simulink model "motor_control_with_homebrew_SVPWM"  (Simulink 7.9)
settings: Solver=ode45  StartTime=0.0  StopTime=1  RelTol=1e-3
libraries: powerlib x17, simulink x6
settings Model: Creator=Dmitriy  LastModifiedBy=Dmitriy
settings GRTTargetCC: CombineOutputUpdateFcns=off  GRTInterface=on

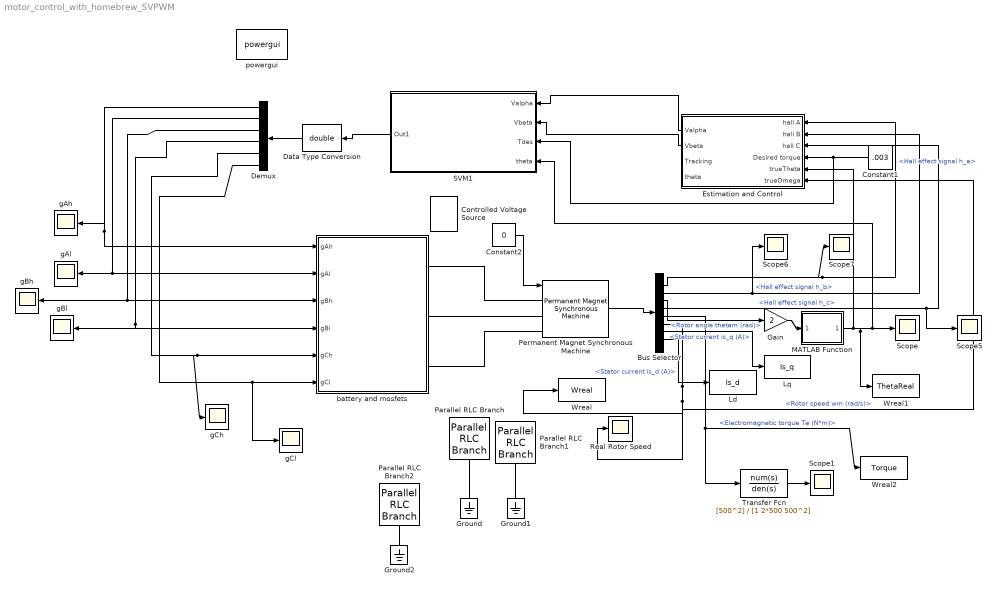
== system motor_control_with_homebrew_SVPWM ==
  Bus Selector : BusSelector  OutputSignals=Hall effect signal h_a,Hall effect signal h_b,Hall effect signal h_c,Rotor angle thetam (rad),Electromagnetic torque Te (N*m),Rotor speed wm (rad/s),Stator current is_q (A),Stator current is_d (A)
  Constant1 : Constant  Value=.003
  Constant2 : Constant  Value=0
  Controlled Voltage Source : powerlib/Electrical Sources/Controlled Voltage Source  Initialize=on  Source_Type=AC  Amplitude=0  Phase=0  Frequency=0  Measurements=None
  Data Type Conversion : DataTypeConversion  OutDataTypeStr=double
  Demux : Demux  Outputs=6
  Estimation and Control : Subsystem  SystemSampleTime=.001
  Gain : Gain  Gain=2
  Ground : powerlib/Elements/Ground  LConnTagsString=a
  Ground1 : powerlib/Elements/Ground  LConnTagsString=a
  Ground2 : powerlib/Elements/Ground  LConnTagsString=a
  Ld : ToWorkspace  VariableName=Is_d  SampleTime=-1  SaveFormat=Timeseries
  Lq : ToWorkspace  VariableName=Is_q  SampleTime=-1  SaveFormat=Timeseries
  MATLAB Function : MATLAB Function  TreatAsAtomicUnit=on
  Parallel RLC Branch : powerlib/Elements/Parallel RLC Branch  LConnTagsString=a  RConnTagsString=__new0  BranchType=RC  Resistance=100000  Inductance=1e-3  SetiL0=off  InitialCurrent=0  Capacitance=1e-4  Setx0=off  InitialVoltage=0  Measurements=None
  Parallel RLC Branch1 : powerlib/Elements/Parallel RLC Branch  LConnTagsString=a  RConnTagsString=__new0  BranchType=RC  Resistance=100000  Inductance=1e-3  SetiL0=off  InitialCurrent=0  Capacitance=1e-4  Setx0=off  InitialVoltage=0  Measurements=None
  Parallel RLC Branch2 : powerlib/Elements/Parallel RLC Branch  LConnTagsString=a  RConnTagsString=__new0  BranchType=RC  Resistance=100000  Inductance=1e-3  SetiL0=off  InitialCurrent=0  Capacitance=1e-4  Setx0=off  InitialVoltage=0  Measurements=None
  Permanent Magnet Synchronous Machine : powerlib/Machines/Permanent Magnet Synchronous Machine  NbPhases=3  FluxDistribution=Sinusoidal  RotorType=Round  MechanicalLoad=Torque Tm  PresetModel=No  ShowDetailedParameters=on  Resistance=28.2  Inductance=8.5e-3  dqInductances=[0.006365 0.006365]  La=1940*10^-6  MachineConstant=Torque Constant (N.m / A_peak)  Flux=0.005225  VoltageCst=1.8954  TorqueCst=0.0181*sqrt(3)/2  Flat=120  Mechanical=[0.0001 5.396e-005 2 0]  PolePairs=2  InitialConditions=[0,1, 0,0]  InitialConditions5ph=[0 0 0 0 0 0]  TsPowergui=0  TsBlock=-1  RefAngle=Aligned with phase A axis (original Park)
  Real Rotor Speed : Scope
      settings: YMin=9.27  YMax=9.44  SaveName=ScopeData18
  SVM1 : Subsystem  SystemSampleTime=10^-6
  Scope{,1,5..7} (5 alike) : Scope
      Scope settings: YMin=0.03925  YMax=0.0396
      Scope1 settings: YMin=0.0028  YMax=0.003275
      Scope5 settings: SaveName=ScopeData5
      Scope6 settings: SaveName=ScopeData6
      Scope7 settings: SaveName=ScopeData7
  Transfer Fcn : TransferFcn  Numerator=[500^2]  Denominator=[1 2*500 500^2]
  Wreal : ToWorkspace  VariableName=Wreal  SampleTime=-1  SaveFormat=Timeseries
  Wreal1 : ToWorkspace  VariableName=ThetaReal  SampleTime=-1  SaveFormat=Timeseries
  Wreal2 : ToWorkspace  VariableName=Torque  SampleTime=-1  SaveFormat=Timeseries
  battery and mosfets : Subsystem
  gAh : Scope
      settings: SaveName=ScopeData11
  gAl : Scope
      settings: SaveName=ScopeData10
  gBh : Scope
      settings: SaveName=ScopeData9
  gBl : Scope
      settings: YMin=0.998725  YMax=0.99925  SaveName=ScopeData8
  gCh : Scope
      settings: YMin=0.95  YMax=1.05  SaveName=ScopeData4
  gCl : Scope
      settings: YMin=0.95  YMax=1.05  SaveName=ScopeData2
  powergui : powerlib/powergui  Priority=1  SimulationMode=Discrete  SolverType=Tustin  SampleTime=1e-6  frequency=60  SPID=off  DisableSnubberDevices=off  DisableRonSwitches=off  DisableVfSwitches=off  SwTol=0  Interpol=off  DisplayEquations=off  FunctionMessages=off  frequencyindice=0  Pbase=100e6  ErrMax=1e-4  Iterations=50  UnitsV=kV  UnitsW=MW  echomessages=off  HookPort=off  EnableUseOfTLC=off  x0status=blocks  RestoreLinks=warning  ResistiveCurrentMeasurement=off  Ylog=off  Xlog=on  ShowGrid=off  save=off  variable=ZData  ZoomFFT=off  StartTime=0.0  cycles=1  DisplayStyle=1  FreqAxis=off  MaxFrequency=1000  frequencyindicesteady=1  display=off  methode=off
  wires:
  Permanent Magnet Synchronous Machine/1 -> Bus Selector/1
  Bus Selector/1 -> Estimation and Control/1(hall A), Scope7/1  "<Hall effect signal h_a>"
  Bus Selector/3 -> Estimation and Control/3(hall C), Scope5/1  "<Hall effect signal h_c>"
  Bus Selector/4 -> Gain/1  "<Rotor angle thetam (rad)>"
  Bus Selector/5 -> Wreal2/1, Transfer Fcn/1  "<Electromagnetic torque Te (N*m)>"
  Bus Selector/2 -> Estimation and Control/2(hall B), Scope6/1  "<Hall effect signal h_b>"
  Demux/6 -> battery and mosfets/6(gCl), gCl/1
  Demux/5 -> battery and mosfets/5(gCh), gCh/1
  Demux/4 -> battery and mosfets/4(gBl), gBl/1
  Demux/3 -> battery and mosfets/3(gBh), gBh/1
  Demux/2 -> battery and mosfets/2(gAl), gAl/1
  Demux/1 -> battery and mosfets/1(gAh), gAh/1
  Constant1/1 -> Estimation and Control/4(Desired torque), SVM1/3(Tdes)
  Bus Selector/6 -> Real Rotor Speed/1, Wreal/1, Estimation and Control/6(trueOmega)  "<Rotor speed wm (rad/s)>"
  MATLAB Function/1(lambda1) -> Wreal1/1, Scope/1, SVM1/4(theta), Estimation and Control/5(trueTheta)
  Gain/1 -> MATLAB Function/1(lambda)
  Constant2/1 -> Permanent Magnet Synchronous Machine/1
  Estimation and Control/1(Valpha) -> SVM1/1(Valpha)
  Estimation and Control/2(Vbeta) -> SVM1/2(Vbeta)
  SVM1/1(Out1) -> Data Type Conversion/1
  Bus Selector/7 -> Lq/1  "<Stator current is_q (A)>"
  Bus Selector/8 -> Ld/1  "<Stator current is_d (A)>"
  Transfer Fcn/1 -> Scope1/1
  Data Type Conversion/1 -> Demux/1
  connections:
  Permanent Magnet Synchronous Machine/LConn1 -- battery and mosfets/RConn1
  battery and mosfets/RConn2 -- Permanent Magnet Synchronous Machine/LConn2
  Permanent Magnet Synchronous Machine/LConn3 -- battery and mosfets/RConn3
  Parallel RLC Branch/RConn1 -- Ground/LConn1
  Ground1/LConn1 -- Parallel RLC Branch1/RConn1
  Parallel RLC Branch2/RConn1 -- Ground2/LConn1

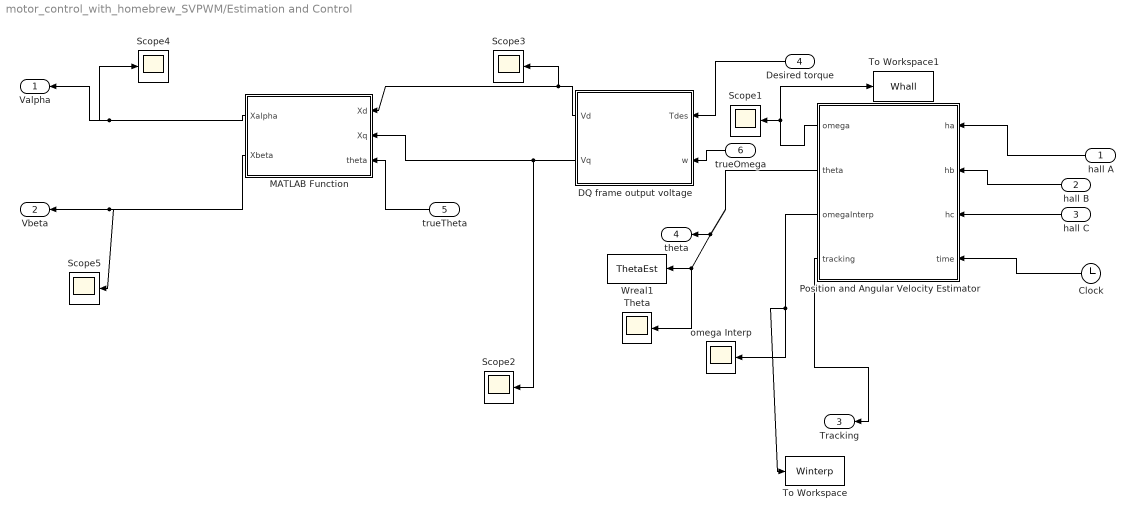
== system motor_control_with_homebrew_SVPWM/Estimation and Control ==
  hall A : Inport
  hall B : Inport  Port=2
  hall C : Inport  Port=3
  Desired torque : Inport  Port=4
  trueTheta : Inport  Port=5
  trueOmega : Inport  Port=6
  Clock : Clock
  DQ frame output voltage : MATLAB Function  TreatAsAtomicUnit=on  SystemSampleTime=.0001
  MATLAB Function : MATLAB Function  TreatAsAtomicUnit=on
  Position and Angular Velocity Estimator : MATLAB Function  TreatAsAtomicUnit=on  SystemSampleTime=.0001
  Scope{1..5} (5 alike) : Scope
      Scope1 settings: SaveName=ScopeData13
      Scope2 settings: YMin=4.67403  YMax=4.67403  SaveName=ScopeData14
      Scope3 settings: SaveName=ScopeData15
      Scope4 settings: SaveName=ScopeData16
      Scope5 settings: SaveName=ScopeData17
  Theta : Scope
      settings: YMin=5.75959  YMax=5.75959  SaveName=ScopeData12
  To Workspace : ToWorkspace  VariableName=Winterp  SampleTime=-1  SaveFormat=Timeseries
  To Workspace1 : ToWorkspace  VariableName=Whall  SampleTime=-1  SaveFormat=Timeseries
  Wreal1 : ToWorkspace  VariableName=ThetaEst  SampleTime=-1  SaveFormat=Timeseries
  omega Interp : Scope
      settings: YMin=0  YMax=3.25  SaveName=ScopeData19
  Valpha : Outport
  Vbeta : Outport  Port=2
  Tracking : Outport  Port=3
  theta : Outport  Port=4
  wires:
  Position and Angular Velocity Estimator/1(omega) -> Scope1/1, To Workspace1/1
  Desired torque/1 -> DQ frame output voltage/1(Tdes)
  hall A/1 -> Position and Angular Velocity Estimator/1(ha)
  hall B/1 -> Position and Angular Velocity Estimator/2(hb)
  hall C/1 -> Position and Angular Velocity Estimator/3(hc)
  Position and Angular Velocity Estimator/2(theta) -> Theta/1, Wreal1/1, theta/1
  DQ frame output voltage/2(Vq) -> Scope2/1, MATLAB Function/2(Xq)
  DQ frame output voltage/1(Vd) -> Scope3/1, MATLAB Function/1(Xd)
  MATLAB Function/1(Xalpha) -> Valpha/1, Scope4/1
  MATLAB Function/2(Xbeta) -> Vbeta/1, Scope5/1
  Position and Angular Velocity Estimator/3(omegaInterp) -> omega Interp/1, To Workspace/1
  Clock/1 -> Position and Angular Velocity Estimator/4(time)
  Position and Angular Velocity Estimator/4(tracking) -> Tracking/1
  trueTheta/1 -> MATLAB Function/3(theta)
  trueOmega/1 -> DQ frame output voltage/2(w)

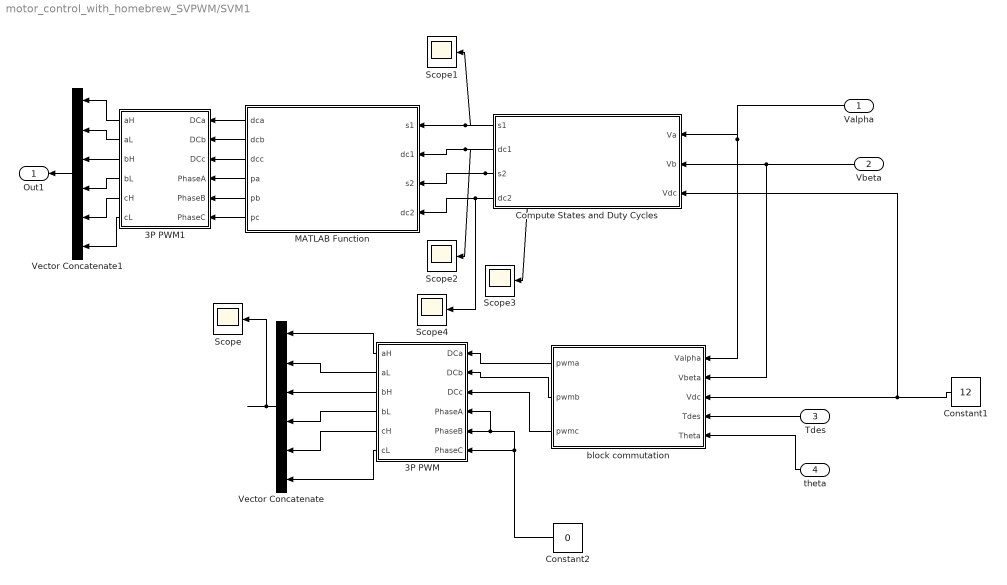
== system motor_control_with_homebrew_SVPWM/SVM1 ==
  Valpha : Inport
  Vbeta : Inport  Port=2
  Tdes : Inport  Port=3
  theta : Inport  Port=4
  3P PWM : Subsystem  TreatAsAtomicUnit=on  SystemSampleTime=1
  3P PWM1 : Subsystem  TreatAsAtomicUnit=on  SystemSampleTime=10^-6
  Compute States and Duty Cycles : MATLAB Function  TreatAsAtomicUnit=on  SystemSampleTime=.001
  Constant1 : Constant  Value=12
  Constant2 : Constant  Value=0
  MATLAB Function : MATLAB Function  TreatAsAtomicUnit=on  SystemSampleTime=10^-6
  Scope{,1..4} (5 alike) : Scope
      Scope settings: SaveName=ScopeData3
      Scope1 settings: SaveName=ScopeData6
      Scope2 settings: SaveName=ScopeData7
      Scope3 settings: SaveName=ScopeData8
      Scope4 settings: SaveName=ScopeData9
  Vector Concatenate : Concatenate  NumInputs=6
  Vector Concatenate1 : Concatenate  NumInputs=6
  block commutation : MATLAB Function  TreatAsAtomicUnit=on  SystemSampleTime=1
  Out1 : Outport
  wires:
  Valpha/1 -> block commutation/1(Valpha), Compute States and Duty Cycles/1(Va)
  Vbeta/1 -> block commutation/2(Vbeta), Compute States and Duty Cycles/2(Vb)
  Constant1/1 -> block commutation/3(Vdc), Compute States and Duty Cycles/3(Vdc)
  Tdes/1 -> block commutation/4(Tdes)
  theta/1 -> block commutation/5(Theta)
  block commutation/2(pwmb) -> 3P PWM/2(DCb)
  block commutation/3(pwmc) -> 3P PWM/3(DCc)
  block commutation/1(pwma) -> 3P PWM/1(DCa)
  3P PWM/1(aH) -> Vector Concatenate/1
  3P PWM/2(aL) -> Vector Concatenate/2
  3P PWM/3(bH) -> Vector Concatenate/3
  3P PWM/4(bL) -> Vector Concatenate/4
  3P PWM/5(cH) -> Vector Concatenate/5
  3P PWM/6(cL) -> Vector Concatenate/6
  Vector Concatenate/1 -> Scope/1
  Constant2/1 -> 3P PWM/6(PhaseC), 3P PWM/5(PhaseB), 3P PWM/4(PhaseA)
  MATLAB Function/1(dca) -> 3P PWM1/1(DCa)
  MATLAB Function/2(dcb) -> 3P PWM1/2(DCb)
  MATLAB Function/3(dcc) -> 3P PWM1/3(DCc)
  MATLAB Function/4(pa) -> 3P PWM1/4(PhaseA)
  MATLAB Function/5(pb) -> 3P PWM1/5(PhaseB)
  MATLAB Function/6(pc) -> 3P PWM1/6(PhaseC)
  3P PWM1/1(aH) -> Vector Concatenate1/1
  3P PWM1/2(aL) -> Vector Concatenate1/2
  3P PWM1/3(bH) -> Vector Concatenate1/3
  3P PWM1/4(bL) -> Vector Concatenate1/4
  3P PWM1/5(cH) -> Vector Concatenate1/5
  3P PWM1/6(cL) -> Vector Concatenate1/6
  Compute States and Duty Cycles/1(s1) -> MATLAB Function/1(s1), Scope1/1
  Compute States and Duty Cycles/2(dc1) -> MATLAB Function/2(dc1), Scope2/1
  Compute States and Duty Cycles/3(s2) -> MATLAB Function/3(s2), Scope3/1
  Compute States and Duty Cycles/4(dc2) -> MATLAB Function/4(dc2), Scope4/1
  Vector Concatenate1/1 -> Out1/1

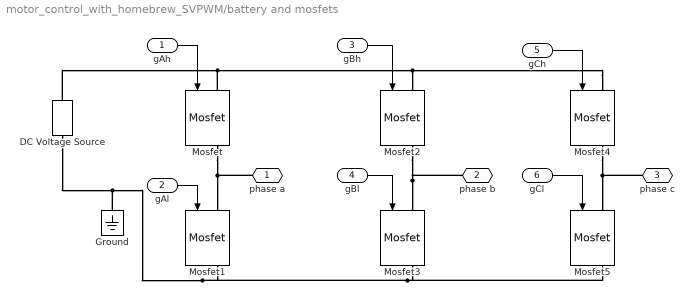
== system motor_control_with_homebrew_SVPWM/battery and mosfets ==
  gAh : Inport
  gAl : Inport  Port=2
  gBh : Inport  Port=3
  gBl : Inport  Port=4
  gCh : Inport  Port=5
  gCl : Inport  Port=6
  DC Voltage Source : powerlib/Electrical Sources/DC Voltage Source  Amplitude=12  Measurements=None
  Ground : powerlib/Elements/Ground  LConnTagsString=a
  Mosfet{,1..5} (6 alike) : powerlib/Power Electronics/Mosfet  Ron=0.1  Lon=0  Rd=0.01  Vfd=0  IC=0  Rs=1e5  Cs=inf  Measurements=on
  phase a : PMIOPort  Port=1  Side=Right
  phase b : PMIOPort  Port=2  Side=Right
  phase c : PMIOPort  Port=3  Side=Right
  wires:
  gCl/1 -> Mosfet5/1
  gCh/1 -> Mosfet4/1
  gBh/1 -> Mosfet2/1
  gBl/1 -> Mosfet3/1
  gAl/1 -> Mosfet1/1
  gAh/1 -> Mosfet/1
  connections:
  Mosfet/RConn1 -- Mosfet1/LConn1 -- phase a/RConn1
  Mosfet2/RConn1 -- Mosfet3/LConn1 -- phase b/RConn1
  phase c/RConn1 -- Mosfet4/RConn1 -- Mosfet5/LConn1
  Mosfet1/RConn1 -- Ground/LConn1 -- DC Voltage Source/LConn1 -- Mosfet3/RConn1 -- Mosfet5/RConn1
  Mosfet4/LConn1 -- Mosfet/LConn1 -- DC Voltage Source/RConn1 -- Mosfet2/LConn1

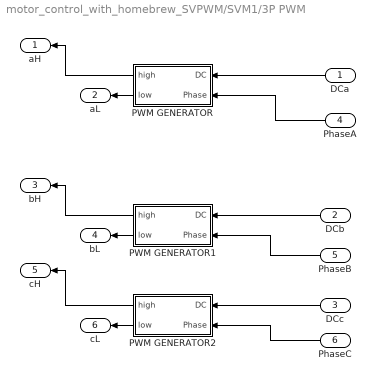
== system motor_control_with_homebrew_SVPWM/SVM1/3P PWM ==
  DCa : Inport
  DCb : Inport  Port=2
  DCc : Inport  Port=3
  PhaseA : Inport  Port=4
  PhaseB : Inport  Port=5
  PhaseC : Inport  Port=6
  PWM GENERATOR : Subsystem  TreatAsAtomicUnit=on
      settings: ErrorFcn=10^6
  PWM GENERATOR1 : Subsystem  TreatAsAtomicUnit=on
  PWM GENERATOR2 : Subsystem  TreatAsAtomicUnit=on
  aH : Outport
  aL : Outport  Port=2
  bH : Outport  Port=3
  bL : Outport  Port=4
  cH : Outport  Port=5
  cL : Outport  Port=6
  wires:
  DCa/1 -> PWM GENERATOR/1(DC)
  PWM GENERATOR/1(high) -> aH/1
  PWM GENERATOR/2(low) -> aL/1
  DCb/1 -> PWM GENERATOR1/1(DC)
  PWM GENERATOR1/1(high) -> bH/1
  PWM GENERATOR1/2(low) -> bL/1
  DCc/1 -> PWM GENERATOR2/1(DC)
  PWM GENERATOR2/1(high) -> cH/1
  PWM GENERATOR2/2(low) -> cL/1
  PhaseA/1 -> PWM GENERATOR/2(Phase)
  PhaseB/1 -> PWM GENERATOR1/2(Phase)
  PhaseC/1 -> PWM GENERATOR2/2(Phase)

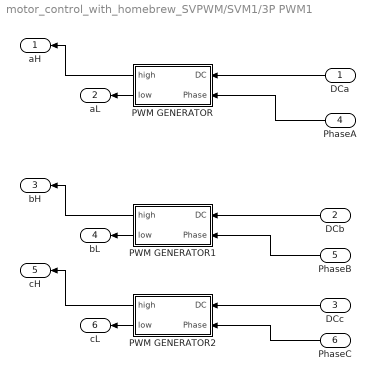
== system motor_control_with_homebrew_SVPWM/SVM1/3P PWM1 ==
  DCa : Inport
  DCb : Inport  Port=2
  DCc : Inport  Port=3
  PhaseA : Inport  Port=4
  PhaseB : Inport  Port=5
  PhaseC : Inport  Port=6
  PWM GENERATOR : Subsystem  TreatAsAtomicUnit=on
      settings: ErrorFcn=10^6
  PWM GENERATOR1 : Subsystem  TreatAsAtomicUnit=on
  PWM GENERATOR2 : Subsystem  TreatAsAtomicUnit=on
  aH : Outport
  aL : Outport  Port=2
  bH : Outport  Port=3
  bL : Outport  Port=4
  cH : Outport  Port=5
  cL : Outport  Port=6
  wires:
  DCa/1 -> PWM GENERATOR/1(DC)
  PWM GENERATOR/1(high) -> aH/1
  PWM GENERATOR/2(low) -> aL/1
  DCb/1 -> PWM GENERATOR1/1(DC)
  PWM GENERATOR1/1(high) -> bH/1
  PWM GENERATOR1/2(low) -> bL/1
  DCc/1 -> PWM GENERATOR2/1(DC)
  PWM GENERATOR2/1(high) -> cH/1
  PWM GENERATOR2/2(low) -> cL/1
  PhaseA/1 -> PWM GENERATOR/2(Phase)
  PhaseB/1 -> PWM GENERATOR1/2(Phase)
  PhaseC/1 -> PWM GENERATOR2/2(Phase)

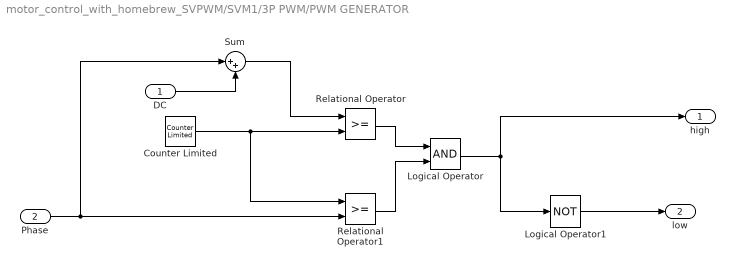
== system motor_control_with_homebrew_SVPWM/SVM1/3P PWM/PWM GENERATOR ==
  DC : Inport
  Phase : Inport  Port=2
  Counter Limited : simulink/Sources/Counter Limited  uplimit=1000  tsamp=-1
  Logical Operator : Logic  AllPortsSameDT=off  OutDataTypeStr=boolean
  Logical Operator1 : Logic  Operator=NOT  AllPortsSameDT=off  OutDataTypeStr=boolean
  Relational Operator : RelationalOperator  OutDataTypeStr=boolean
  Relational Operator1 : RelationalOperator  OutDataTypeStr=boolean
  Sum : Sum  Inputs=|++
  high : Outport
  low : Outport  Port=2
  wires:
  Counter Limited/1 -> Relational Operator/2, Relational Operator1/1
  Phase/1 -> Relational Operator1/2, Sum/1
  DC/1 -> Sum/2
  Sum/1 -> Relational Operator/1
  Relational Operator/1 -> Logical Operator/1
  Relational Operator1/1 -> Logical Operator/2
  Logical Operator/1 -> Logical Operator1/1, high/1
  Logical Operator1/1 -> low/1

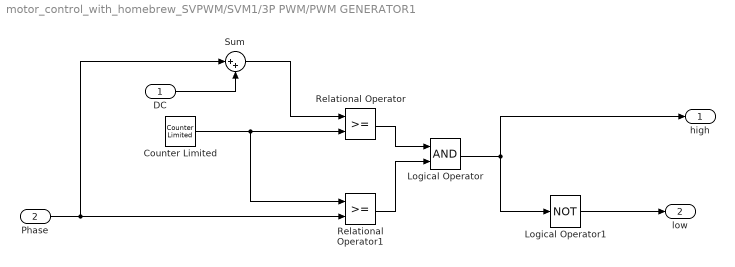
== system motor_control_with_homebrew_SVPWM/SVM1/3P PWM/PWM GENERATOR1 ==
  DC : Inport
  Phase : Inport  Port=2
  Counter Limited : simulink/Sources/Counter Limited  uplimit=1000  tsamp=-1
  Logical Operator : Logic  AllPortsSameDT=off  OutDataTypeStr=boolean
  Logical Operator1 : Logic  Operator=NOT  AllPortsSameDT=off  OutDataTypeStr=boolean
  Relational Operator : RelationalOperator  OutDataTypeStr=boolean
  Relational Operator1 : RelationalOperator  OutDataTypeStr=boolean
  Sum : Sum  Inputs=|++
  high : Outport
  low : Outport  Port=2
  wires:
  Counter Limited/1 -> Relational Operator/2, Relational Operator1/1
  Phase/1 -> Relational Operator1/2, Sum/1
  DC/1 -> Sum/2
  Sum/1 -> Relational Operator/1
  Relational Operator/1 -> Logical Operator/1
  Relational Operator1/1 -> Logical Operator/2
  Logical Operator/1 -> Logical Operator1/1, high/1
  Logical Operator1/1 -> low/1

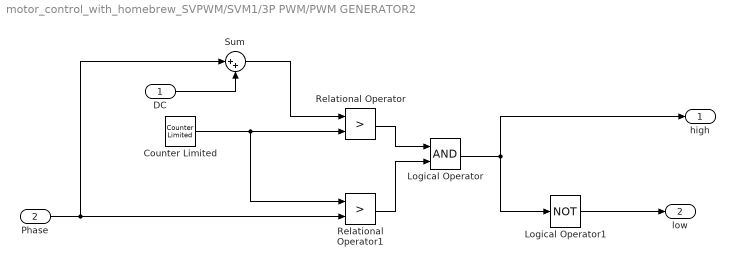
== system motor_control_with_homebrew_SVPWM/SVM1/3P PWM/PWM GENERATOR2 ==
  DC : Inport
  Phase : Inport  Port=2
  Counter Limited : simulink/Sources/Counter Limited  uplimit=1000  tsamp=-1
  Logical Operator : Logic  AllPortsSameDT=off  OutDataTypeStr=boolean
  Logical Operator1 : Logic  Operator=NOT  AllPortsSameDT=off  OutDataTypeStr=boolean
  Relational Operator : RelationalOperator  Operator=>  OutDataTypeStr=boolean
  Relational Operator1 : RelationalOperator  Operator=>  OutDataTypeStr=boolean
  Sum : Sum  Inputs=|++
  high : Outport
  low : Outport  Port=2
  wires:
  Counter Limited/1 -> Relational Operator/2, Relational Operator1/1
  Phase/1 -> Relational Operator1/2, Sum/1
  DC/1 -> Sum/2
  Sum/1 -> Relational Operator/1
  Relational Operator/1 -> Logical Operator/1
  Relational Operator1/1 -> Logical Operator/2
  Logical Operator/1 -> Logical Operator1/1, high/1
  Logical Operator1/1 -> low/1

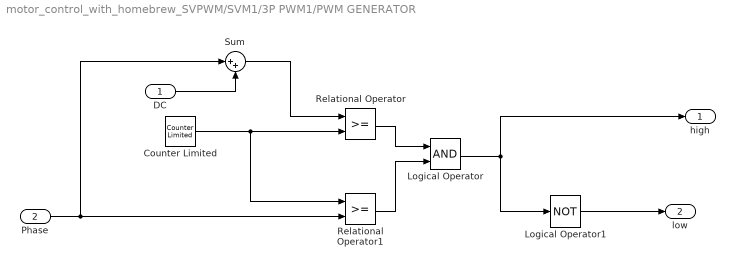
== system motor_control_with_homebrew_SVPWM/SVM1/3P PWM1/PWM GENERATOR ==
  DC : Inport
  Phase : Inport  Port=2
  Counter Limited : simulink/Sources/Counter Limited  uplimit=1000  tsamp=-1
  Logical Operator : Logic  AllPortsSameDT=off  OutDataTypeStr=boolean
  Logical Operator1 : Logic  Operator=NOT  AllPortsSameDT=off  OutDataTypeStr=boolean
  Relational Operator : RelationalOperator  OutDataTypeStr=boolean
  Relational Operator1 : RelationalOperator  OutDataTypeStr=boolean
  Sum : Sum  Inputs=|++
  high : Outport
  low : Outport  Port=2
  wires:
  Counter Limited/1 -> Relational Operator/2, Relational Operator1/1
  Phase/1 -> Relational Operator1/2, Sum/1
  DC/1 -> Sum/2
  Sum/1 -> Relational Operator/1
  Relational Operator/1 -> Logical Operator/1
  Relational Operator1/1 -> Logical Operator/2
  Logical Operator/1 -> Logical Operator1/1, high/1
  Logical Operator1/1 -> low/1

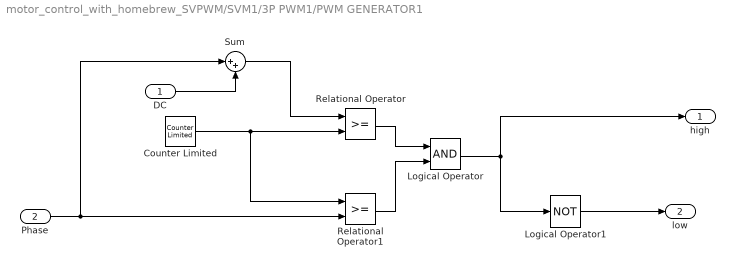
== system motor_control_with_homebrew_SVPWM/SVM1/3P PWM1/PWM GENERATOR1 ==
  DC : Inport
  Phase : Inport  Port=2
  Counter Limited : simulink/Sources/Counter Limited  uplimit=1000  tsamp=-1
  Logical Operator : Logic  AllPortsSameDT=off  OutDataTypeStr=boolean
  Logical Operator1 : Logic  Operator=NOT  AllPortsSameDT=off  OutDataTypeStr=boolean
  Relational Operator : RelationalOperator  OutDataTypeStr=boolean
  Relational Operator1 : RelationalOperator  OutDataTypeStr=boolean
  Sum : Sum  Inputs=|++
  high : Outport
  low : Outport  Port=2
  wires:
  Counter Limited/1 -> Relational Operator/2, Relational Operator1/1
  Phase/1 -> Relational Operator1/2, Sum/1
  DC/1 -> Sum/2
  Sum/1 -> Relational Operator/1
  Relational Operator/1 -> Logical Operator/1
  Relational Operator1/1 -> Logical Operator/2
  Logical Operator/1 -> Logical Operator1/1, high/1
  Logical Operator1/1 -> low/1

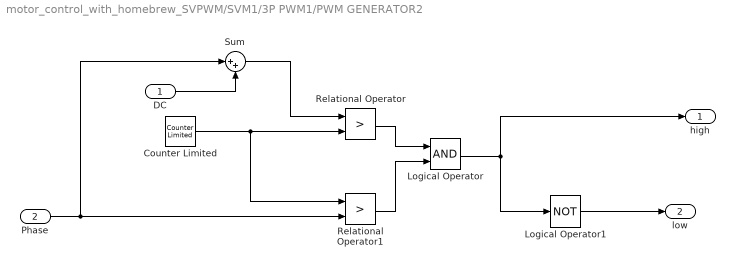
== system motor_control_with_homebrew_SVPWM/SVM1/3P PWM1/PWM GENERATOR2 ==
  DC : Inport
  Phase : Inport  Port=2
  Counter Limited : simulink/Sources/Counter Limited  uplimit=1000  tsamp=-1
  Logical Operator : Logic  AllPortsSameDT=off  OutDataTypeStr=boolean
  Logical Operator1 : Logic  Operator=NOT  AllPortsSameDT=off  OutDataTypeStr=boolean
  Relational Operator : RelationalOperator  Operator=>  OutDataTypeStr=boolean
  Relational Operator1 : RelationalOperator  Operator=>  OutDataTypeStr=boolean
  Sum : Sum  Inputs=|++
  high : Outport
  low : Outport  Port=2
  wires:
  Counter Limited/1 -> Relational Operator/2, Relational Operator1/1
  Phase/1 -> Relational Operator1/2, Sum/1
  DC/1 -> Sum/2
  Sum/1 -> Relational Operator/1
  Relational Operator/1 -> Logical Operator/1
  Relational Operator1/1 -> Logical Operator/2
  Logical Operator/1 -> Logical Operator1/1, high/1
  Logical Operator1/1 -> low/1

== matlab function Estimation and Control/DQ frame output voltage ==
  data: Tdes input double; Vd output double; w input double; Vq output double
function [Vd,Vq] = computeDQOutput(Tdes,w)
%#codegen
%take the desired torque current 
% speed and compute the output voltage vector in the DQ
%frame. 

L = 1940*10^-6*sqrt(3)/2;
R = 28.2;
Ke = (1.895*10^-3)*9.54929659643; % convert to V/(rad/s) 
Kt = 18.1*10^-3*sqrt(3)/2; %Nm/Amp
Ke = Kt;

%because I is assumed to be on Q axis, T = KtI
Ides = Tdes/Kt

%bemf is on q axis
bemf = Ke*w

%inductor impedance 
ZL = L*w;

Vq = (bemf+Ides*R)*3/2
Vd = (-ZL*Ides)*3/2

== matlab function Estimation and Control/Position and Angular Velocity Estimator ==
  data: omega output double; ha input double; theta output double; hb input double; hc input double; omegaInterp output double; time input double; tracking output double
function [omega,theta, omegaInterp, tracking] = rotor_est(ha,hb,hc,time)
%#codegen

%estimate the position of the rotor in degrees electrical
%tracking is 0 or 1, 0 means the estimate is bad. Used for activating block
%commutation at initialization
omega=0;
theta=0;
omegaInterp = 0;
time
tracking =0;
coder.extrinsic('rotor_estimate');

[omega theta omegaInterp tracking] = rotor_estimate(ha,hb,hc,time);
end

== matlab function MATLAB Function ==
  data: lambda input double; lambda1 output double
function lambda1 = wrapTo2Pi(lambda)
%wrapTo2Pi Wrap angle in radians to [0 2*pi]
%
%   lambdaWrapped = wrapTo2Pi(LAMBDA) wraps angles in LAMBDA, in radians,
%   to the interval [0 2*pi] such that zero maps to zero and 2*pi maps
%   to 2*pi. (In general, positive multiples of 2*pi map to 2*pi and
%   negative multiples of 2*pi map to zero.)
%
%   See also wrapToPi, wrapTo180, wrapTo360.

% Copyright 2007-2008 The MathWorks, Inc.
% $Revision: 1.1.6.1 $  $Date: 2008/12/22 23:50:53 $


positiveInput = (lambda > 0);
lambda = mod(lambda, 2*pi);
lambda((lambda == 0) & positiveInput) = 2*pi;
lambda1=lambda;
end

== matlab function Estimation and Control/MATLAB Function ==
  data: Xd input double; Xalpha output double; Xq input double; theta input double; Xbeta output double
function [Xalpha,Xbeta] = inversePark(Xd,Xq,theta)
%#codegen
%implements inverse park as described in james mevey's thesis

c = cos(theta);
s = sin(theta);

ipm = [c -s; s c];

xab = ipm*[Xd Xq]';

Xalpha = xab(1);
Xbeta = xab(2);
end

== matlab function SVM1/Compute States and Duty Cycles ==
  data: Va input double; s1 output double; dc1 output double; Vb input double; s2 output double; Vdc input double; dc2 output double
function [s1,dc1, s2, dc2] = statesAndCycles(Va,Vb, Vdc)
%#codegen
    %Given desired Valpha and Vbeta, and the supply voltage, compute the inverter states to toggle
    %between and the duty cycle of each
    
    %right now we're saying that the length of each state vector is Vdc, which
    %is probably wrong
    
    ang = wrapTo2Pi(angle(Va+1i*Vb));
    
    sext = floor(ang/(pi/3))
    
    v1 = 1 +1i;
    v2 = 1 + 1i;
    
    %states as defined in james mevey's thesis
    %v1, v2 are complex values of the voltages
    switch sext
        case 0
            s1 = 1;
            v1 = Vdc;
            
            s2 = 2;
            [t1 t2] = pol2cart(pi/3,Vdc);
            v2 = t1+1i*t2;
            
        case 1
            s1 = 2;
            [t1 t2] = pol2cart(pi/3,Vdc);
            v1 = t1+1i*t2;
            
            s2 = 3;
            [t1 t2] = pol2cart(2*pi/3,Vdc);
            v2 = t1+1i*t2;
            
        case 2
            s1 = 3;
            [t1 t2] = pol2cart(2*pi/3,Vdc);
            v1 = t1+1i*t2;
            
            s2 = 4;
            [t1 t2] = pol2cart(pi,Vdc);
            v2 = t1+1i*t2;
        case 3
            s1 = 4;
            [t1 t2] = pol2cart(pi,Vdc);
            v1 = t1+1i*t2;
            
            s2 = 5;
            [t1 t2] = pol2cart(4*pi/3,Vdc);
            v2 = t1+1i*t2;
        case 4
            s1 = 5;
            [t1 t2] = pol2cart(4*pi/3,Vdc);
            v1 = t1+1i*t2;
            
            
            s2 = 6;
            [t1 t2] = pol2cart(5*pi/3,Vdc);
            v2 = t1+1i*t2;
        case 5
            s1 = 6;
            [t1 t2] = pol2cart(5*pi/3,Vdc);
            v1 = t1+1i*t2;
            
            s2 = 1;
            v2 = Vdc;
        otherwise
            s1 = 0;
            s2 = 0;
    end
    
v1 
v2
num = Vb - imag(v1)*Va/real(v1)
den = imag(v2)-imag(v1)*real(v2)/real(v1)
dc2 = num/den;
dc1 = (Va - real(v2)*dc2)/real(v1);


    %solve for intersection of v1 line and v2 line translated to the desired
    %place
    
% 
%     num = Va-imag(v2)*Vb/real(v2)- imag(v1);
%     den = real(v1) - imag(v2)/real(v2);
%     
%     xint = num/den;
%     yint = (imag(v1)/real(v1))*xint;
%     
%     %duty cycle 1 equals length of sv1 divided by Vdc, which is nominal length
%     dc1 = sqrt(xint^2+yint^2)/Vdc;
%     
%     %duty cycle 2 is distance from the tip of sv1 to the desired point, divided
%     %by Vdc
%     
%     dc2 = sqrt((xint-Va)^2 +(yint - Vb)^2)/Vdc;

end

function lambda = wrapTo2Pi(lambda)
%wrapTo2Pi Wrap angle in radians to [0 2*pi]
%
%   lambdaWrapped = wrapTo2Pi(LAMBDA) wraps angles in LAMBDA, in radians,
%   to the interval [0 2*pi] such that zero maps to zero and 2*pi maps
%   to 2*pi. (In general, positive multiples of 2*pi map to 2*pi and
%   negative multiples of 2*pi map to zero.)
%
%   See also wrapToPi, wrapTo180, wrapTo360.

% Copyright 2007-2008 The MathWorks, Inc.
% $Revision: 1.1.6.1 $  $Date: 2008/12/22 23:50:53 $

positiveInput = (lambda > 0);
lambda = mod(lambda, 2*pi);
lambda((lambda == 0) & positiveInput) = 2*pi;
end

function p = angle(h)
%ANGLE  Phase angle.
%   ANGLE(H) returns the phase angles, in radians, of a matrix with
%   complex elements.
%
%   Class support for input X:
%      float: double, single
%
%   See also ABS, UNWRAP.

%   Copyright 1984-2010 The MathWorks, Inc.
%   $Revision: 5.7.4.2 $  $Date: 2010/04/21 21:31:19 $

p = atan2(imag(h), real(h));
end

== matlab function SVM1/MATLAB Function ==
  data: s1 input double; dca output double; dc1 input double; s2 input double; dc2 input double; dcb output double; dcc output double; pa output double; pb output double; pc output double
function [dca,dcb,dcc,pa,pb,pc] = PWM_module_inputs(s1,dc1,s2,dc2)
%#codegen
%given the two states to switch between and the duty cycle of each, compute
%the proper duty cycles and phases for each leg of the half bridge. Duty
%cycles should be between 1 and 1000, as should phases. If duty cycle is
%1000, and phase is 400, then the duty cycle really only ends up being 400,
%get it? If not, look at the pwm block.

%pattern is: all low, then s1, then s2

d1 = dc1*1000;
d2 = dc2*1000;
p2 = 1000-d2;
d0 = 1000 - d1 -d2;
p0 = 0;
p1 = d0;

dca = 1000;
dcb = 1000;
dcc = 1000;

switch(s1)
    
    case 1
        pa = d0;
        if(s2==2)
            pb = d0+d1;
            pc = 1000;
        else
            pb = 1000;
            pc = d0+d1;
        end
    case 2
        pc = 1000;
        if(s2==3)
            dca = d1;
            pa = d0;
            pb = d0;
        else
            pa = d0;
            dcb = d1;
            pb = d0;
        end
    case 3
        pb = d0;
        if(s2==4)
            pa = 1000;
            pc = d0+d1;
        else
            pa = d0+d1;
            pc =1000;
        end
    case 4
        pa = 1000;
        if(s2 == 5)
            dcb = d1;
            pb = d0;
            pc = d0;
        else
            pb = d0;
            dcc = d1;
            pc = d0;
        end
    case 5
        pc = d0;
        if(s2==6)
            pa = d0+d1;
            pb = 1000;
        else
            pa = 1000;
            pb = d0+d1;
        end
    case 6
        pb=1000;
        if(s2==1)
            pa = d0;
            dcc = d1;
            pc = d0;
        else
            dca = d1;
            pa = d0;
            pc = d0;
        end
    otherwise
        pa=1000;
        pb = 1000;
        pc = 1000;
end

end

== matlab function SVM1/block commutation ==
  data: Valpha input double; pwma output double; Vbeta input double; Vdc input double; Tdes input double; Theta input double; pwmb output double; pwmc output double
function [pwma,pwmb,pwmc]  = block_com(Valpha,Vbeta,Vdc,Tdes,Theta)
%#codegen

ang = floor(Theta/(pi/3));

d = sqrt(Valpha^2+Vbeta^2)/Vdc;
d = 1;


switch ang
    case 0
        if(Tdes>=0)
            %s2
            pwms = [d d 0];
        else
            %s1
            pwms = [d 0 0];
        end
    case 1
        if(Tdes>=0)
            %s3
            pwms = [0 d 0];
        else
            %s2
            pwms = [d d 0];
        end
        
    case 2
        if(Tdes>=0)
            %s4
            pwms = [0 d d];
        else
            %s3
            pwms = [0 d 0];
        end
    case 3
        if(Tdes>=0)
            %s5
            pwms = [0 0 d];
        else
            %s4
            pwms = [0 d d];
        end
    case 4
        if(Tdes>=0)
            %s6
            pwms = [d 0 d];
        else
            %s5
            pwms = [0 0 d];
        end
    case 5
        if(Tdes>=0)
            %s1
            pwms = [d 0 0];
        else
            %s6
            pwms = [d 0 d];
        end
        
    otherwise
        pwms = [0 0 0];
end
pwms=pwms*1000;
pwma=pwms(1);
pwmb= pwms(2);
pwmc = pwms(3);
